simulink library "ammclib_bam_S32K3xx"  (R2016a)
(part 27 of 50)

      |           warning('Natural frequency f0 must be positive.');
      |         end
      |         if (iksi<=0)
      |           warning('Current loop attenuation must be positive.');
      |         end
      |         if (iksi>1)
      |           warning('Current loop attenuation must not exceed 1.');
      |         end
      |         pgain=12.56637061435917*iksi*if0;
      |         igain=39.47841760435743*if0*if0;
      |         if strcmp(intmethod,'Forward Rectangular')
      |           cc1=pgain;
      |           cc2=-pgain+igain*SampleTime;
      |         else
      |           if strcmp(intmethod,'Backward Rectangular')
      |             cc1=pgain+igain*SampleTime;
      |             cc2=-pgain;
      |           else
      |             cc1=pgain+igain*SampleTime*0.5;
      |             cc2=-pgain+igain*SampleTime*0.5;
      |           end
      |         end
      |         fltCC1sc=cc1;
      |         fltCC2sc=cc2;
      |         fltLowerLimit=-1000000.0;
      |         fltUpperLimit=1000000.0;
      |         fltC1=SampleTime*0.5;
      |         if isnan(fltCC1sc)
      |           if ~strcmp(fltCC1sc_bkup,'0')
      |             set_param(gcb,'fltCC1sc','0');
      |           end
      |         else
      |           tmps=num2str(fltCC1sc);
      |           if ~strcmp(fltCC1sc_bkup,tmps)
      |             set_param(gcb,'fltCC1sc',tmps);
      |           end
      |         end
      |         if isnan(fltCC2sc)
      |           if ~strcmp(fltCC2sc_bkup,'0')
      |             set_param(gcb,'fltCC2sc','0');
      |           end
      |         else
      |           tmps=num2str(fltCC2sc);
      |           if ~strcmp(fltCC2sc_bkup,tmps)
      |             set_param(gcb,'fltCC2sc',tmps);
      |           end
      |         end
      |         if isnan(fltUpperLimit)
      |           if ~strcmp(fltUpperLimit_bkup,'0')
      |             set_param(gcb,'fltUpperLimit','0');
      |           end
      |         else
      |           tmps=num2str(fltUpperLimit);
      |           if ~strcmp(fltUpperLimit_bkup,tmps)
      |             set_param(gcb,'fltUpperLimit',tmps);
      |           end
      |         end
      |         if isnan(fltLowerLimit)
      |           if ~strcmp(fltLowerLimit_bkup,'0')
      |             set_param(gcb,'fltLowerLimit','0');
      |           end
      |         else
      |           tmps=num2str(fltLowerLimit);
      |           if ~strcmp(fltLowerLimit_bkup,tmps)
      |             set_param(gcb,'fltLowerLimit',tmps);
      |           end
      |         end
      |         if isnan(fltC1)
      |           if ~strcmp(fltC1_bkup,'0')
      |             set_param(gcb,'fltC1','0');
      |           end
      |         else
      |           tmps=num2str(fltC1);
      |           if ~strcmp(fltC1_bkup,tmps)
      |             set_param(gcb,'fltC1',tmps);
      |           end
      |         end
      |       end
      |     end
      |   catch
      |    warning(['Sample time cannot be calculated for the block ' gcb])
      |   end
      | end
      mask DialogControl timeHint Prompt: Note: Implementation parameters cannot be calculated yet because the block's inherited sample time is unknown. Simulink will update the sample time when you run the simulation.
      mask Display:
      | color('black');
      | pos = get_param(gcb, 'Position');
      | width = pos(3) - pos(1);
      | height = pos(4) - pos(2);
      | tX=width/2;
      | tY=height - 25;
      | color('black');
      | text(tX,tY, 'AMCLIB_TrackObsrv_FLT', 'horizontalAlignment', 'center');
      | if showStates == 2
      |   color('red');
      |   text(tX,tY - 20, ['debugging mode' char(13) char(10) '(limited performance)'], 'horizontalAlignment', 'center');
      | end
  AMCLIB_Windmilling_FLT : Subsystem  StartFcn=|  TreatAsAtomicUnit=on  mask(AMCLIB_Windmilling_FLT){showStates=Hide (faster execution), SampleTime=-1, if0=350, iksi=1, ADCMaxError=0.002, autoCalcEn=on, fltADCMaxError=0, fltCC1sc=0, fltCC2sc=0, fltUpperLimit=0, fltLowerLimit=0, fltC1=0, SampleTime_1=NaN}
      | ts=get_param(gcb,'CompiledSampleTime');
      | if iscell(ts)
      |   ts=ts{1};
      |   if iscell(ts)
      |     ts=ts{1};
      |   end
      | end
      | ts=ts(1);
      | set_param(gcb,'SampleTime_1',num2str(ts));
      | p=Simulink.Mask.get(gcb);
      | hintText=p.getDialogControl('timeHint');
      | SampleTime=Simulink.data.evalinGlobal(bdroot,get_param(gcb,'SampleTime'));
      | p=Simulink.Mask.get(gcb);
      | autoCalcEn=get_param(gcb,'autoCalcEn');
      | if strcmp(autoCalcEn,'on')
      |   if SampleTime==-1
      |     hintText.Prompt='Caution: Implementation parameters depend on inherited sample time. Make sure that the sample time of the block''s inputs corresponds to the sampling period in the target application.';
      |   else
      |     hintText.Prompt='Caution: Implementation parameters depend on the sample time. Make sure that the simulation time step corresponds to the sampling period in the target application.';
      |   end
      |   SampleTime=ts;
      |   fltADCMaxError_bkup=get_param(gcb,'fltADCMaxError');
      |   fltCC1sc_bkup=get_param(gcb,'fltCC1sc');
      |   fltCC2sc_bkup=get_param(gcb,'fltCC2sc');
      |   fltUpperLimit_bkup=get_param(gcb,'fltUpperLimit');
      |   fltLowerLimit_bkup=get_param(gcb,'fltLowerLimit');
      |   fltC1_bkup=get_param(gcb,'fltC1');
      |   if0=Simulink.data.evalinGlobal(bdroot,get_param(gcb,'if0'));
      |   iksi=Simulink.data.evalinGlobal(bdroot,get_param(gcb,'iksi'));
      |   ADCMaxError=Simulink.data.evalinGlobal(bdroot,get_param(gcb,'ADCMaxError'));
      |   if (if0<=0)
      |     warning('Natural frequency f0 must be positive.');
      |   end
      |   if (iksi<=0)
      |     warning('Feedback loop attenuation must be positive.');
      |   end
      |   if (iksi>1)
      |     warning('Feedback loop attenuation must not exceed 1.');
      |   end
      |   if (ADCMaxError<=0)
      |     warning('fltADCMaxError must be positive.');
      |   end
      |   fltADCMaxError=ADCMaxError;
      |   pgain=12.56637061435917*iksi*if0;
      |   igain=39.47841760435743*if0*if0;
      |   cc1=pgain+igain*SampleTime*0.5;
      |   cc2=-pgain+igain*SampleTime*0.5;
      |   fltCC1sc=cc1;
      |   fltCC2sc=cc2;
      |   fltLowerLimit=-1000000.0;
      |   fltUpperLimit=1000000.0;
      |   fltC1=SampleTime*0.5;
      |   if isnan(fltADCMaxError)
      |     if ~strcmp(fltADCMaxError_bkup,'0')
      |       set_param(gcb,'fltADCMaxError','0');
      |     end
      |   else
      |     tmps=num2str(fltADCMaxError);
      |     if ~strcmp(fltADCMaxError_bkup,tmps)
      |       set_param(gcb,'fltADCMaxError',tmps);
      |     end
      |   end
      |   if isnan(fltCC1sc)
      |     if ~strcmp(fltCC1sc_bkup,'0')
      |       set_param(gcb,'fltCC1sc','0');
      |     end
      |   else
      |     tmps=num2str(fltCC1sc);
      |     if ~strcmp(fltCC1sc_bkup,tmps)
      |       set_param(gcb,'fltCC1sc',tmps);
      |     end
      |   end
      |   if isnan(fltCC2sc)
      |     if ~strcmp(fltCC2sc_bkup,'0')
      |       set_param(gcb,'fltCC2sc','0');
      |     end
      |   else
      |     tmps=num2str(fltCC2sc);
      |     if ~strcmp(fltCC2sc_bkup,tmps)
      |       set_param(gcb,'fltCC2sc',tmps);
      |     end
      |   end
      |   if isnan(fltUpperLimit)
      |     if ~strcmp(fltUpperLimit_bkup,'0')
      |       set_param(gcb,'fltUpperLimit','0');
      |     end
      |   else
      |     tmps=num2str(fltUpperLimit);
      |     if ~strcmp(fltUpperLimit_bkup,tmps)
      |       set_param(gcb,'fltUpperLimit',tmps);
      |     end
      |   end
      |   if isnan(fltLowerLimit)
      |     if ~strcmp(fltLowerLimit_bkup,'0')
      |       set_param(gcb,'fltLowerLimit','0');
      |     end
      |   else
      |     tmps=num2str(fltLowerLimit);
      |     if ~strcmp(fltLowerLimit_bkup,tmps)
      |       set_param(gcb,'fltLowerLimit',tmps);
      |     end
      |   end
      |   if isnan(fltC1)
      |     if ~strcmp(fltC1_bkup,'0')
      |       set_param(gcb,'fltC1','0');
      |     end
      |   else
      |     tmps=num2str(fltC1);
      |     if ~strcmp(fltC1_bkup,tmps)
      |       set_param(gcb,'fltC1',tmps);
      |     end
      |   end
      | end
      mask prompts: showStates "Show internal states:"; SampleTime "Sample time (-1 for inherited):"; if0 "Feedback loop natural frequency f0 [Hz]:"; iksi "Feedback loop attenuation ξ:"; ADCMaxError "Maximum differential offset error between any two
phases of the 3-phase voltage-sensing A/D converters [V]:"; autoCalcEn "Calculate implementation parameters from physical parameters"; fltADCMaxError "fltADCMaxError (Max. ADC differential offset error):"; fltCC1sc "fltCC1sc (GFLIB_ControllerPIrAW - CC1 coefficient):"; fltCC2sc "fltCC2sc (GFLIB_ControllerPIrAW - CC2 coefficient):"; fltUpperLimit "fltUpperLimit (GFLIB_ControllerPIrAW - upper Limit of the controller):"; fltLowerLimit "fltLowerLimit (GFLIB_ControllerPIrAW - lower Limit of the controller):"; fltC1 "fltC1 (GFLIB_IntegratorTR - integrator coefficient):"; SampleTime_1 "Discrete sample time:"
      mask help: PMSM Windmilling in single precision floating-point implementation. This function detects spontaneous rotation of an unpowered 3-phase PMSM by measuring the generated back electromotive force. Output u32Lock represents the return value of the C function (0 = undecided, 1 = spinning, 2 = stopped). Transition from 0 to 1 on the u32Lock output can be taken as a reset signal for the following AMCLIB_TrackObsrv_FLT block to synchronize the sensorless FOC loop with a freewheeling motor. Refer to the AMMCLIB User's Guide for further details.
      mask init:
      | ddName = get_param(bdroot,'DataDictionary');
      | if length(ddName)==0
      |   set_param(bdroot,'DataDictionary','ammclib_types.sldd');
      | else
      |   dd = Simulink.data.dictionary.open(ddName);
      |   data = getSection(dd,'Design Data');
      |   if ~exist(data,'SWLIBS_2Syst_F16')
      |     addDataSource(dd,'ammclib_types.sldd');
      |     saveChanges(dd);
      |   end
      | end
      | 
      | if showStates == 1
      |   % hidden state variables
      |   if strcmp(get_param([gcb '/fltADCMaxError'], 'BlockType'), 'Inport')
      |     posblk = get_param(gcb, 'Position');
      | 
      |     pos = get_param([gcb, '/fltADCMaxError'], 'Position');
      |     orient = get_param([gcb, '/fltADCMaxError'], 'Orientation');
      |     delete_block([gcb, '/fltADCMaxError']);
      |     add_block('built-in/Ground', [gcb, '/fltADCMaxError'], 'Position', pos, 'Orientation', orient);
      | 
      |     pos = get_param([gcb, '/fltCC1sc'], 'Position');
      |     orient = get_param([gcb, '/fltCC1sc'], 'Orientation');
      |     delete_block([gcb, '/fltCC1sc']);
      |     add_block('built-in/Ground', [gcb, '/fltCC1sc'], 'Position', pos, 'Orientation', orient);
      | 
      |     pos = get_param([gcb, '/fltCC2sc'], 'Position');
      |     orient = get_param([gcb, '/fltCC2sc'], 'Orientation');
      |     delete_block([gcb, '/fltCC2sc']);
      |     add_block('built-in/Ground', [gcb, '/fltCC2sc'], 'Position', pos, 'Orientation', orient);
      | 
      |     pos = get_param([gcb, '/fltUpperLimit'], 'Position');
      |     orient = get_param([gcb, '/fltUpperLimit'], 'Orientation');
      |     delete_block([gcb, '/fltUpperLimit']);
      |     add_block('built-in/Ground', [gcb, '/fltUpperLimit'], 'Position', pos, 'Orientation', orient);
      | 
      |     pos = get_param([gcb, '/fltLowerLimit'], 'Position');
      |     orient = get_param([gcb, '/fltLowerLimit'], 'Orientation');
      |     delete_block([gcb, '/fltLowerLimit']);
      |     add_block('built-in/Ground', [gcb, '/fltLowerLimit'], 'Position', pos, 'Orientation', orient);
      | 
      |     pos = get_param([gcb, '/fltC1'], 'Position');
      |     orient = get_param([gcb, '/fltC1'], 'Orientation');
      |     delete_block([gcb, '/fltC1']);
      |     add_block('built-in/Ground', [gcb, '/fltC1'], 'Position', pos, 'Orientation', orient);
      | 
      |     pos = get_param([gcb, '/fltAccPI'], 'Position');
      |     orient = get_param([gcb, '/fltAccPI'], 'Orientation');
      |     delete_block([gcb, '/fltAccPI']);
      |     add_block('built-in/Ground', [gcb, '/fltAccPI'], 'Position', pos, 'Orientation', orient);
      | 
      |     pos = get_param([gcb, '/fltInErrK1'], 'Position');
      |     orient = get_param([gcb, '/fltInErrK1'], 'Orientation');
      |     delete_block([gcb, '/fltInErrK1']);
      |     add_block('built-in/Ground', [gcb, '/fltInErrK1'], 'Position', pos, 'Orientation', orient);
      | 
      |     pos = get_param([gcb, '/fltState'], 'Position');
      |     orient = get_param([gcb, '/fltState'], 'Orientation');
      |     delete_block([gcb, '/fltState']);
      |     add_block('built-in/Ground', [gcb, '/fltState'], 'Position', pos, 'Orientation', orient);
      | 
      |     pos = get_param([gcb, '/fltInK1'], 'Position');
      |     orient = get_param([gcb, '/fltInK1'], 'Orientation');
      |     delete_block([gcb, '/fltInK1']);
      |     add_block('built-in/Ground', [gcb, '/fltInK1'], 'Position', pos, 'Orientation', orient);
      | 
      | 
      |     pmask=Simulink.Mask.get(gcb);
      |     pctrl=pmask.getParameter('SampleTime');
      |     pctrl.set('TypeOptions',{'pUabcIn/SampleTime'});
      | 
      |     pos = get_param([gcb '/fltAccPI_Out'], 'Position');
      |     orient = get_param([gcb '/fltAccPI_Out'], 'Orientation');
      |     delete_block([gcb '/fltAccPI_Out']);
      |     add_block('built-in/Terminator', [gcb '/fltAccPI_Out'], 'Position', pos, 'Orientation', orient);
      | 
      |     pos = get_param([gcb '/fltInErrK1_Out'], 'Position');
      |     orient = get_param([gcb '/fltInErrK1_Out'], 'Orientation');
      |     delete_block([gcb '/fltInErrK1_Out']);
      |     add_block('built-in/Terminator', [gcb '/fltInErrK1_Out'], 'Position', pos, 'Orientation', orient);
      | 
      |     pos = get_param([gcb '/fltState_Out'], 'Position');
      |     orient = get_param([gcb '/fltState_Out'], 'Orientation');
      |     delete_block([gcb '/fltState_Out']);
      |     add_block('built-in/Terminator', [gcb '/fltState_Out'], 'Position', pos, 'Orientation', orient);
      | 
      |     pos = get_param([gcb '/fltInK1_Out'], 'Position');
      |     orient = get_param([gcb '/fltInK1_Out'], 'Orientation');
      |     delete_block([gcb '/fltInK1_Out']);
      |     add_block('built-in/Terminator', [gcb '/fltInK1_Out'], 'Position', pos, 'Orientation', orient);
      | 
      |     set_param([gcb '/pUabcIn'], 'Port', '1');
      | 
      |     tmpOutCnt=0;
      |     tmpOutCnt=tmpOutCnt+1;
      |     set_param([gcb '/u32Lock'], 'Port', num2str(tmpOutCnt));
      |     tmpOutCnt=tmpOutCnt+1;
      |     set_param([gcb '/pPosEst'], 'Port', num2str(tmpOutCnt));
      |     tmpOutCnt=tmpOutCnt+1;
      |     set_param([gcb '/pVelocityEst'], 'Port', num2str(tmpOutCnt));
      | 
      |     autoCalcEn=get_param(gcb,'autoCalcEn');
      |     if strcmp(autoCalcEn,'on')
      |       set_param(gcb,'MaskEnables',{'on','on','on','on','on','on','on','on','on','on','on','on','off'});
      |     else
      |       set_param(gcb,'MaskEnables',{'on','on','off','off','off','on','on','on','on','on','on','on','off'});
      |     end
      | 
      |     if (posblk(4) - posblk(2)) > 100
      |       height = 100;
      |       set_param(gcb,'Position',[posblk(1), posblk(2), posblk(3), posblk(2)+height])
      |     end
      |   end
      | else
      |   % shown state variables
      |   if strcmp(get_param([gcb '/fltADCMaxError'], 'BlockType'), 'Ground')
      |     posblk = get_param(gcb, 'Position');
      | 
      |     pos = get_param([gcb, '/fltADCMaxError'], 'Position');
      |     orient = get_param([gcb, '/fltADCMaxError'], 'Orientation');
      |     delete_block([gcb, '/fltADCMaxError']);
      |     add_block('built-in/Inport', [gcb, '/fltADCMaxError'], 'Position', pos, 'Orientation', orient, 'OutDataTypeStr', 'single');
      | 
      |     pos = get_param([gcb, '/fltCC1sc'], 'Position');
      |     orient = get_param([gcb, '/fltCC1sc'], 'Orientation');
      |     delete_block([gcb, '/fltCC1sc']);
      |     add_block('built-in/Inport', [gcb, '/fltCC1sc'], 'Position', pos, 'Orientation', orient, 'OutDataTypeStr', 'single');
      | 
      |     pos = get_param([gcb, '/fltCC2sc'], 'Position');
      |     orient = get_param([gcb, '/fltCC2sc'], 'Orientation');
      |     delete_block([gcb, '/fltCC2sc']);
      |     add_block('built-in/Inport', [gcb, '/fltCC2sc'], 'Position', pos, 'Orientation', orient, 'OutDataTypeStr', 'single');
      | 
      |     pos = get_param([gcb, '/fltUpperLimit'], 'Position');
      |     orient = get_param([gcb, '/fltUpperLimit'], 'Orientation');
      |     delete_block([gcb, '/fltUpperLimit']);
      |     add_block('built-in/Inport', [gcb, '/fltUpperLimit'], 'Position', pos, 'Orientation', orient, 'OutDataTypeStr', 'single');
      | 
      |     pos = get_param([gcb, '/fltLowerLimit'], 'Position');
      |     orient = get_param([gcb, '/fltLowerLimit'], 'Orientation');
      |     delete_block([gcb, '/fltLowerLimit']);
      |     add_block('built-in/Inport', [gcb, '/fltLowerLimit'], 'Position', pos, 'Orientation', orient, 'OutDataTypeStr', 'single');
      | 
      |     pos = get_param([gcb, '/fltC1'], 'Position');
      |     orient = get_param([gcb, '/fltC1'], 'Orientation');
      |     delete_block([gcb, '/fltC1']);
      |     add_block('built-in/Inport', [gcb, '/fltC1'], 'Position', pos, 'Orientation', orient, 'OutDataTypeStr', 'single');
      | 
      |     pos = get_param([gcb, '/fltAccPI'], 'Position');
      |     orient = get_param([gcb, '/fltAccPI'], 'Orientation');
      |     delete_block([gcb, '/fltAccPI']);
      |     add_block('built-in/Inport', [gcb, '/fltAccPI'], 'Position', pos, 'Orientation', orient, 'OutDataTypeStr', 'single');
      | 
      |     pos = get_param([gcb, '/fltInErrK1'], 'Position');
      |     orient = get_param([gcb, '/fltInErrK1'], 'Orientation');
      |     delete_block([gcb, '/fltInErrK1']);
      |     add_block('built-in/Inport', [gcb, '/fltInErrK1'], 'Position', pos, 'Orientation', orient, 'OutDataTypeStr', 'single');
      | 
      |     pos = get_param([gcb, '/fltState'], 'Position');
      |     orient = get_param([gcb, '/fltState'], 'Orientation');
      |     delete_block([gcb, '/fltState']);
      |     add_block('built-in/Inport', [gcb, '/fltState'], 'Position', pos, 'Orientation', orient, 'OutDataTypeStr', 'single');
      | 
      |     pos = get_param([gcb, '/fltInK1'], 'Position');
      |     orient = get_param([gcb, '/fltInK1'], 'Orientation');
      |     delete_block([gcb, '/fltInK1']);
      |     add_block('built-in/Inport', [gcb, '/fltInK1'], 'Position', pos, 'Orientation', orient, 'OutDataTypeStr', 'single');
      | 
      | 
      | 
      |     pos = get_param([gcb '/fltAccPI_Out'], 'Position');
      |     orient = get_param([gcb '/fltAccPI_Out'], 'Orientation');
      |     delete_block([gcb '/fltAccPI_Out']);
      |     add_block('built-in/Outport', [gcb '/fltAccPI_Out'], 'Position', pos, 'Orientation', orient);
      | 
      |     pos = get_param([gcb '/fltInErrK1_Out'], 'Position');
      |     orient = get_param([gcb '/fltInErrK1_Out'], 'Orientation');
      |     delete_block([gcb '/fltInErrK1_Out']);
      |     add_block('built-in/Outport', [gcb '/fltInErrK1_Out'], 'Position', pos, 'Orientation', orient);
      | 
      |     pos = get_param([gcb '/fltState_Out'], 'Position');
      |     orient = get_param([gcb '/fltState_Out'], 'Orientation');
      |     delete_block([gcb '/fltState_Out']);
      |     add_block('built-in/Outport', [gcb '/fltState_Out'], 'Position', pos, 'Orientation', orient);
      | 
      |     pos = get_param([gcb '/fltInK1_Out'], 'Position');
      |     orient = get_param([gcb '/fltInK1_Out'], 'Orientation');
      |     delete_block([gcb '/fltInK1_Out']);
      |     add_block('built-in/Outport', [gcb '/fltInK1_Out'], 'Position', pos, 'Orientation', orient);
      | 
      | 
      |     pmask=Simulink.Mask.get(gcb);
      |     pctrl=pmask.getParameter('SampleTime');
      |     pctrl.set('TypeOptions',{'pUabcIn/SampleTime','fltADCMaxError/SampleTime','fltCC1sc/SampleTime','fltCC2sc/SampleTime','fltUpperLimit/SampleTime','fltLowerLimit/SampleTime','fltC1/SampleTime','fltAccPI/SampleTime','fltInErrK1/SampleTime','fltState/SampleTime','fltInK1/SampleTime'});
      | 
      |     set_param([gcb '/pUabcIn'], 'Port', '1');
      |     set_param([gcb '/fltADCMaxError'], 'Port', '2');
      |     set_param([gcb '/fltCC1sc'], 'Port', '3');
      |     set_param([gcb '/fltCC2sc'], 'Port', '4');
      |     set_param([gcb '/fltUpperLimit'], 'Port', '5');
      |     set_param([gcb '/fltLowerLimit'], 'Port', '6');
      |     set_param([gcb '/fltC1'], 'Port', '7');
      |     set_param([gcb '/fltAccPI'], 'Port', '8');
      |     set_param([gcb '/fltInErrK1'], 'Port', '9');
      |     set_param([gcb '/fltState'], 'Port', '10');
      |     set_param([gcb '/fltInK1'], 'Port', '11');
      | 
      |     tmpOutCnt=0;
      |     tmpOutCnt=tmpOutCnt+1;
      |     set_param([gcb '/u32Lock'], 'Port', num2str(tmpOutCnt));
      |     tmpOutCnt=tmpOutCnt+1;
      |     set_param([gcb '/pPosEst'], 'Port', num2str(tmpOutCnt));
      |     tmpOutCnt=tmpOutCnt+1;
      |     set_param([gcb '/pVelocityEst'], 'Port', num2str(tmpOutCnt));
      |     tmpOutCnt=tmpOutCnt+1;
      |     set_param([gcb '/fltAccPI_Out'], 'Port', num2str(tmpOutCnt));
      |     tmpOutCnt=tmpOutCnt+1;
      |     set_param([gcb '/fltInErrK1_Out'], 'Port', num2str(tmpOutCnt));
      |     tmpOutCnt=tmpOutCnt+1;
      |     set_param([gcb '/fltState_Out'], 'Port', num2str(tmpOutCnt));
      |     tmpOutCnt=tmpOutCnt+1;
      |     set_param([gcb '/fltInK1_Out'], 'Port', num2str(tmpOutCnt));
      | 
      |     set_param(gcb,'MaskEnables',{'on','on','off','off','off','off','off','off','off','off','off','off','off'});
      | 
      |     if (posblk(4) - posblk(2)) < 300
      |       height = 300;
      |       set_param(gcb,'Position',[posblk(1), posblk(2), posblk(3), posblk(2)+height])
      |     end
      |   end
      | end
      settings: RTWSystemCode=Inline
      mask Help: web([fileparts(which('ammclib_bam_S32K3xx.slx')) '/../doc/S32K3XXMCLUG.pdf'], '-browser')
      mask TypeOptions showStates: Hide (faster execution) | Show (allows debugging; connect feedback loops manually)
      mask Callback showStates:
      | maskStr=get_param(gcb,'showStates');
      | if strcmp(maskStr,'Hide (faster execution)')
      |   if strcmp(get_param([gcb '/fltADCMaxError'], 'BlockType'), 'Inport')
      |     autoCalcEn=get_param(gcb,'autoCalcEn');
      |     if strcmp(autoCalcEn,'on')
      |       set_param(gcb,'MaskEnables',{'on','on','on','on','on','on','on','on','on','on','on','on','off'});
      |     else
      |       set_param(gcb,'MaskEnables',{'on','on','off','off','off','on','on','on','on','on','on','on','off'});
      |     end
      |   end
      | else
      |   if strcmp(get_param([gcb '/fltADCMaxError'], 'BlockType'), 'Ground')
      |     set_param(gcb,'MaskEnables',{'on','on','off','off','off','off','off','off','off','off','off','off','off'});
      |   end
      | end
      mask TypeOptions SampleTime: pUabcIn/SampleTime
      mask Callback SampleTime:
      | p=Simulink.Mask.get(gcb);
      | hintText=p.getDialogControl('timeHint');
      | SampleTime=Simulink.data.evalinGlobal(bdroot,get_param(gcb,'SampleTime'));
      | SampleTime_1=str2double(get_param(gcb,'SampleTime_1'));
      | if (((SampleTime==-1) && (~contains(hintText.Prompt,'inherited'))) || ...
      |     ((SampleTime~=-1) && contains(hintText.Prompt,'inherited')) || ...
      |     ((SampleTime~=-1) && (SampleTime_1~=SampleTime)) || ...
      |     ((SampleTime_1~=-1) && contains(hintText.Prompt,'yet')))
      |   if ((SampleTime==-1) && (~contains(hintText.Prompt,'inherited')))
      |     set_param(gcb,'SampleTime_1',num2str(NaN));
      |     SampleTime_1=NaN;
      |   end
      |   if (SampleTime~=-1)
      |     set_param(gcb,'SampleTime_1',num2str(SampleTime));
      |     SampleTime_1=SampleTime;
      |   end
      |   autoCalcEn=get_param(gcb,'autoCalcEn');
      |   if strcmp(autoCalcEn,'on')
      |     p=Simulink.Mask.get(gcb);
      |     hintText=p.getDialogControl('timeHint');
      |     if SampleTime==-1
      |       SampleTime=SampleTime_1;
      |       if isnan(SampleTime)
      |         hintText.Prompt='Note: Implementation parameters cannot be calculated yet because the block''s inherited sample time is unknown. Simulink will update the sample time when you run the simulation.';
      |       else
      |         hintText.Prompt='Caution: Implementation parameters depend on inherited sample time. Make sure that the sample time of the block''s inputs corresponds to the sampling period in the target application.';
      |       end
      |     else
      |       hintText.Prompt='Caution: Implementation parameters depend on the sample time. Make sure that the simulation time step corresponds to the sampling period in the target application.';
      |     end
      |     fltADCMaxError_bkup=get_param(gcb,'fltADCMaxError');
      |     fltCC1sc_bkup=get_param(gcb,'fltCC1sc');
      |     fltCC2sc_bkup=get_param(gcb,'fltCC2sc');
      |     fltUpperLimit_bkup=get_param(gcb,'fltUpperLimit');
      |     fltLowerLimit_bkup=get_param(gcb,'fltLowerLimit');
      |     fltC1_bkup=get_param(gcb,'fltC1');
      |     if0=Simulink.data.evalinGlobal(bdroot,get_param(gcb,'if0'));
      |     iksi=Simulink.data.evalinGlobal(bdroot,get_param(gcb,'iksi'));
      |     ADCMaxError=Simulink.data.evalinGlobal(bdroot,get_param(gcb,'ADCMaxError'));
      |     if (if0<=0)
      |       warning('Natural frequency f0 must be positive.');
      |     end
      |     if (iksi<=0)
      |       warning('Feedback loop attenuation must be positive.');
      |     end
      |     if (iksi>1)
      |       warning('Feedback loop attenuation must not exceed 1.');
      |     end
      |     if (ADCMaxError<=0)
      |       warning('fltADCMaxError must be positive.');
      |     end
      |     fltADCMaxError=ADCMaxError;
      |     pgain=12.56637061435917*iksi*if0;
      |     igain=39.47841760435743*if0*if0;
      |     cc1=pgain+igain*SampleTime*0.5;
      |     cc2=-pgain+igain*SampleTime*0.5;
      |     fltCC1sc=cc1;
      |     fltCC2sc=cc2;
      |     fltLowerLimit=-1000000.0;
      |     fltUpperLimit=1000000.0;
      |     fltC1=SampleTime*0.5;
      |     if isnan(fltADCMaxError)
      |       if ~strcmp(fltADCMaxError_bkup,'0')
      |         set_param(gcb,'fltADCMaxError','0');
      |       end
      |     else
      |       tmps=num2str(fltADCMaxError);
      |       if ~strcmp(fltADCMaxError_bkup,tmps)
      |         set_param(gcb,'fltADCMaxError',tmps);
      |       end
      |     end
      |     if isnan(fltCC1sc)
      |       if ~strcmp(fltCC1sc_bkup,'0')
      |         set_param(gcb,'fltCC1sc','0');
      |       end
      |     else
      |       tmps=num2str(fltCC1sc);
      |       if ~strcmp(fltCC1sc_bkup,tmps)
      |         set_param(gcb,'fltCC1sc',tmps);
      |       end
      |     end
      |     if isnan(fltCC2sc)
      |       if ~strcmp(fltCC2sc_bkup,'0')
      |         set_param(gcb,'fltCC2sc','0');
      |       end
      |     else
      |       tmps=num2str(fltCC2sc);
      |       if ~strcmp(fltCC2sc_bkup,tmps)
      |         set_param(gcb,'fltCC2sc',tmps);
      |       end
      |     end
      |     if isnan(fltUpperLimit)
      |       if ~strcmp(fltUpperLimit_bkup,'0')
      |         set_param(gcb,'fltUpperLimit','0');
      |       end
      |     else
      |       tmps=num2str(fltUpperLimit);
      |       if ~strcmp(fltUpperLimit_bkup,tmps)
      |         set_param(gcb,'fltUpperLimit',tmps);
      |       end
      |     end
      |     if isnan(fltLowerLimit)
      |       if ~strcmp(fltLowerLimit_bkup,'0')
      |         set_param(gcb,'fltLowerLimit','0');
      |       end
      |     else
      |       tmps=num2str(fltLowerLimit);
      |       if ~strcmp(fltLowerLimit_bkup,tmps)
      |         set_param(gcb,'fltLowerLimit',tmps);
      |       end
      |     end
      |     if isnan(fltC1)
      |       if ~strcmp(fltC1_bkup,'0')
      |         set_param(gcb,'fltC1','0');
      |       end
      |     else
      |       tmps=num2str(fltC1);
      |       if ~strcmp(fltC1_bkup,tmps)
      |         set_param(gcb,'fltC1',tmps);
      |       end
      |     end
      |   end
      | end
      mask Callback if0:
      | autoCalcEn=get_param(gcb,'autoCalcEn');
      | if strcmp(autoCalcEn,'on')
      |   SampleTime=Simulink.data.evalinGlobal(bdroot,get_param(gcb,'SampleTime'));
      |   if (SampleTime==-1)
      |     SampleTime=str2double(get_param(gcb,'SampleTime_1'));
      |   end
      |   fltADCMaxError_bkup=get_param(gcb,'fltADCMaxError');
      |   fltCC1sc_bkup=get_param(gcb,'fltCC1sc');
      |   fltCC2sc_bkup=get_param(gcb,'fltCC2sc');
      |   fltUpperLimit_bkup=get_param(gcb,'fltUpperLimit');
      |   fltLowerLimit_bkup=get_param(gcb,'fltLowerLimit');
      |   fltC1_bkup=get_param(gcb,'fltC1');
      |   if0=Simulink.data.evalinGlobal(bdroot,get_param(gcb,'if0'));
      |   iksi=Simulink.data.evalinGlobal(bdroot,get_param(gcb,'iksi'));
      |   ADCMaxError=Simulink.data.evalinGlobal(bdroot,get_param(gcb,'ADCMaxError'));
      |   if (if0<=0)
      |     warning('Natural frequency f0 must be positive.');
      |   end
      |   if (iksi<=0)
      |     warning('Feedback loop attenuation must be positive.');
      |   end
      |   if (iksi>1)
      |     warning('Feedback loop attenuation must not exceed 1.');
      |   end
      |   if (ADCMaxError<=0)
      |     warning('fltADCMaxError must be positive.');
      |   end
      |   fltADCMaxError=ADCMaxError;
      |   pgain=12.56637061435917*iksi*if0;
      |   igain=39.47841760435743*if0*if0;
      |   cc1=pgain+igain*SampleTime*0.5;
      |   cc2=-pgain+igain*SampleTime*0.5;
      |   fltCC1sc=cc1;
      |   fltCC2sc=cc2;
      |   fltLowerLimit=-1000000.0;
      |   fltUpperLimit=1000000.0;
      |   fltC1=SampleTime*0.5;
      |   if isnan(fltADCMaxError)
      |     if ~strcmp(fltADCMaxError_bkup,'0')
      |       set_param(gcb,'fltADCMaxError','0');
      |     end
      |   else
      |     tmps=num2str(fltADCMaxError);
      |     if ~strcmp(fltADCMaxError_bkup,tmps)
      |       set_param(gcb,'fltADCMaxError',tmps);
      |     end
      |   end
      |   if isnan(fltCC1sc)
      |     if ~strcmp(fltCC1sc_bkup,'0')
      |       set_param(gcb,'fltCC1sc','0');
      |     end
      |   else
      |     tmps=num2str(fltCC1sc);
      |     if ~strcmp(fltCC1sc_bkup,tmps)
      |       set_param(gcb,'fltCC1sc',tmps);
      |     end
      |   end
      |   if isnan(fltCC2sc)
      |     if ~strcmp(fltCC2sc_bkup,'0')
      |       set_param(gcb,'fltCC2sc','0');
      |     end
      |   else
      |     tmps=num2str(fltCC2sc);
      |     if ~strcmp(fltCC2sc_bkup,tmps)
      |       set_param(gcb,'fltCC2sc',tmps);
      |     end
      |   end
      |   if isnan(fltUpperLimit)
      |     if ~strcmp(fltUpperLimit_bkup,'0')
      |       set_param(gcb,'fltUpperLimit','0');
      |     end
      |   else
      |     tmps=num2str(fltUpperLimit);
      |     if ~strcmp(fltUpperLimit_bkup,tmps)
      |       set_param(gcb,'fltUpperLimit',tmps);
      |     end
      |   end
      |   if isnan(fltLowerLimit)
      |     if ~strcmp(fltLowerLimit_bkup,'0')
      |       set_param(gcb,'fltLowerLimit','0');
      |     end
      |   else
      |     tmps=num2str(fltLowerLimit);
      |     if ~strcmp(fltLowerLimit_bkup,tmps)
      |       set_param(gcb,'fltLowerLimit',tmps);
      |     end
      |   end
      |   if isnan(fltC1)
      |     if ~strcmp(fltC1_bkup,'0')
      |       set_param(gcb,'fltC1','0');
      |     end
      |   else
      |     tmps=num2str(fltC1);
      |     if ~strcmp(fltC1_bkup,tmps)
      |       set_param(gcb,'fltC1',tmps);
      |     end
      |   end
      | end
      mask Callback iksi:
      | autoCalcEn=get_param(gcb,'autoCalcEn');
      | if strcmp(autoCalcEn,'on')
      |   SampleTime=Simulink.data.evalinGlobal(bdroot,get_param(gcb,'SampleTime'));
      |   if (SampleTime==-1)
      |     SampleTime=str2double(get_param(gcb,'SampleTime_1'));
      |   end
      |   fltADCMaxError_bkup=get_param(gcb,'fltADCMaxError');
      |   fltCC1sc_bkup=get_param(gcb,'fltCC1sc');
      |   fltCC2sc_bkup=get_param(gcb,'fltCC2sc');
      |   fltUpperLimit_bkup=get_param(gcb,'fltUpperLimit');
      |   fltLowerLimit_bkup=get_param(gcb,'fltLowerLimit');
      |   fltC1_bkup=get_param(gcb,'fltC1');
      |   if0=Simulink.data.evalinGlobal(bdroot,get_param(gcb,'if0'));
      |   iksi=Simulink.data.evalinGlobal(bdroot,get_param(gcb,'iksi'));
      |   ADCMaxError=Simulink.data.evalinGlobal(bdroot,get_param(gcb,'ADCMaxError'));
      |   if (if0<=0)
      |     warning('Natural frequency f0 must be positive.');
      |   end
      |   if (iksi<=0)
      |     warning('Feedback loop attenuation must be positive.');
      |   end
      |   if (iksi>1)
      |     warning('Feedback loop attenuation must not exceed 1.');
      |   end
      |   if (ADCMaxError<=0)
      |     warning('fltADCMaxError must be positive.');
      |   end
      |   fltADCMaxError=ADCMaxError;
      |   pgain=12.56637061435917*iksi*if0;
      |   igain=39.47841760435743*if0*if0;
      |   cc1=pgain+igain*SampleTime*0.5;
      |   cc2=-pgain+igain*SampleTime*0.5;
      |   fltCC1sc=cc1;
      |   fltCC2sc=cc2;
      |   fltLowerLimit=-1000000.0;
      |   fltUpperLimit=1000000.0;
      |   fltC1=SampleTime*0.5;
      |   if isnan(fltADCMaxError)
      |     if ~strcmp(fltADCMaxError_bkup,'0')
      |       set_param(gcb,'fltADCMaxError','0');
      |     end
      |   else
      |     tmps=num2str(fltADCMaxError);
      |     if ~strcmp(fltADCMaxError_bkup,tmps)
      |       set_param(gcb,'fltADCMaxError',tmps);
      |     end
      |   end
      |   if isnan(fltCC1sc)
      |     if ~strcmp(fltCC1sc_bkup,'0')
      |       set_param(gcb,'fltCC1sc','0');
      |     end
      |   else
      |     tmps=num2str(fltCC1sc);
      |     if ~strcmp(fltCC1sc_bkup,tmps)
      |       set_param(gcb,'fltCC1sc',tmps);
      |     end
      |   end
      |   if isnan(fltCC2sc)
      |     if ~strcmp(fltCC2sc_bkup,'0')
      |       set_param(gcb,'fltCC2sc','0');
      |     end
      |   else
      |     tmps=num2str(fltCC2sc);
      |     if ~strcmp(fltCC2sc_bkup,tmps)
      |       set_param(gcb,'fltCC2sc',tmps);
      |     end
      |   end
      |   if isnan(fltUpperLimit)
      |     if ~strcmp(fltUpperLimit_bkup,'0')
      |       set_param(gcb,'fltUpperLimit','0');
      |     end
      |   else
      |     tmps=num2str(fltUpperLimit);
      |     if ~strcmp(fltUpperLimit_bkup,tmps)
      |       set_param(gcb,'fltUpperLimit',tmps);
      |     end
      |   end
      |   if isnan(fltLowerLimit)
      |     if ~strcmp(fltLowerLimit_bkup,'0')
      |       set_param(gcb,'fltLowerLimit','0');
      |     end
      |   else
      |     tmps=num2str(fltLowerLimit);
      |     if ~strcmp(fltLowerLimit_bkup,tmps)
      |       set_param(gcb,'fltLowerLimit',tmps);
      |     end
      |   end
      |   if isnan(fltC1)
      |     if ~strcmp(fltC1_bkup,'0')
      |       set_param(gcb,'fltC1','0');
      |     end
      |   else
      |     tmps=num2str(fltC1);
      |     if ~strcmp(fltC1_bkup,tmps)
      |       set_param(gcb,'fltC1',tmps);
      |     end
      |   end
      | end
      mask Callback ADCMaxError:
      | autoCalcEn=get_param(gcb,'autoCalcEn');
      | if strcmp(autoCalcEn,'on')
      |   SampleTime=Simulink.data.evalinGlobal(bdroot,get_param(gcb,'SampleTime'));
      |   if (SampleTime==-1)
      |     SampleTime=str2double(get_param(gcb,'SampleTime_1'));
      |   end
      |   fltADCMaxError_bkup=get_param(gcb,'fltADCMaxError');
      |   fltCC1sc_bkup=get_param(gcb,'fltCC1sc');
      |   fltCC2sc_bkup=get_param(gcb,'fltCC2sc');
      |   fltUpperLimit_bkup=get_param(gcb,'fltUpperLimit');
      |   fltLowerLimit_bkup=get_param(gcb,'fltLowerLimit');
      |   fltC1_bkup=get_param(gcb,'fltC1');
      |   if0=Simulink.data.evalinGlobal(bdroot,get_param(gcb,'if0'));
      |   iksi=Simulink.data.evalinGlobal(bdroot,get_param(gcb,'iksi'));
      |   ADCMaxError=Simulink.data.evalinGlobal(bdroot,get_param(gcb,'ADCMaxError'));
      |   if (if0<=0)
      |     warning('Natural frequency f0 must be positive.');
      |   end
      |   if (iksi<=0)
      |     warning('Feedback loop attenuation must be positive.');
      |   end
      |   if (iksi>1)
      |     warning('Feedback loop attenuation must not exceed 1.');
      |   end
      |   if (ADCMaxError<=0)
      |     warning('fltADCMaxError must be positive.');
      |   end
      |   fltADCMaxError=ADCMaxError;
      |   pgain=12.56637061435917*iksi*if0;
      |   igain=39.47841760435743*if0*if0;
      |   cc1=pgain+igain*SampleTime*0.5;
      |   cc2=-pgain+igain*SampleTime*0.5;
      |   fltCC1sc=cc1;
      |   fltCC2sc=cc2;
      |   fltLowerLimit=-1000000.0;
      |   fltUpperLimit=1000000.0;
      |   fltC1=SampleTime*0.5;
      |   if isnan(fltADCMaxError)
      |     if ~strcmp(fltADCMaxError_bkup,'0')
      |       set_param(gcb,'fltADCMaxError','0');
      |     end
      |   else
      |     tmps=num2str(fltADCMaxError);
      |     if ~strcmp(fltADCMaxError_bkup,tmps)
      |       set_param(gcb,'fltADCMaxError',tmps);
      |     end
      |   end
      |   if isnan(fltCC1sc)
      |     if ~strcmp(fltCC1sc_bkup,'0')
      |       set_param(gcb,'fltCC1sc','0');
      |     end
      |   else
      |     tmps=num2str(fltCC1sc);
      |     if ~strcmp(fltCC1sc_bkup,tmps)
      |       set_param(gcb,'fltCC1sc',tmps);
      |     end
      |   end
      |   if isnan(fltCC2sc)
      |     if ~strcmp(fltCC2sc_bkup,'0')
      |       set_param(gcb,'fltCC2sc','0');
      |     end
      |   else
      |     tmps=num2str(fltCC2sc);
      |     if ~strcmp(fltCC2sc_bkup,tmps)
      |       set_param(gcb,'fltCC2sc',tmps);
      |     end
      |   end
      |   if isnan(fltUpperLimit)
      |     if ~strcmp(fltUpperLimit_bkup,'0')
      |       set_param(gcb,'fltUpperLimit','0');
      |     end
      |   else
      |     tmps=num2str(fltUpperLimit);
      |     if ~strcmp(fltUpperLimit_bkup,tmps)
      |       set_param(gcb,'fltUpperLimit',tmps);
      |     end
      |   end
      |   if isnan(fltLowerLimit)
      |     if ~strcmp(fltLowerLimit_bkup,'0')
      |       set_param(gcb,'fltLowerLimit','0');
      |     end
      |   else
      |     tmps=num2str(fltLowerLimit);
      |     if ~strcmp(fltLowerLimit_bkup,tmps)
      |       set_param(gcb,'fltLowerLimit',tmps);
      |     end
      |   end
      |   if isnan(fltC1)
      |     if ~strcmp(fltC1_bkup,'0')
      |       set_param(gcb,'fltC1','0');
      |     end
      |   else
      |     tmps=num2str(fltC1);
      |     if ~strcmp(fltC1_bkup,tmps)
      |       set_param(gcb,'fltC1',tmps);
      |     end
      |   end
      | end
      mask Callback autoCalcEn:
      | maskStr=get_param(gcb,'showStates');
      | if strcmp(maskStr,'Hide (faster execution)')
      |   p=Simulink.Mask.get(gcb);
      |   autoCalcEn=get_param(gcb,'autoCalcEn');
      |   hintText=p.getDialogControl('timeHint');
      |   if strcmp(autoCalcEn,'on')
      |     param=p.getParameter('ADCMaxError');
      |     if strcmp(param.Enabled,'off')
      |       SampleTime=Simulink.data.evalinGlobal(bdroot,get_param(gcb,'SampleTime'));
      |       if SampleTime==-1
      |         SampleTime=str2double(get_param(gcb,'SampleTime_1'));
      |         if isnan(SampleTime)
      |           hintText.Prompt=['Note: Implementation parameters cannot be calculated yet because the block''s inherited sample time is unknown. Simulink will update the sample time when you run the simulation.'];
      |         else
      |           hintText.Prompt=['Caution: Implementation parameters depend on inherited sample time. Make sure that the sample time of the block''s inputs corresponds to the sampling period in the target application.'];
      |         end
      |       else
      |         hintText.Prompt='Caution: Implementation parameters depend on the sample time. Make sure that the simulation time step corresponds to the sampling period in the target application.';
      |       end
      |       p=Simulink.Mask.get(gcb);
      |       param=p.getParameter('if0');
      |       param.set('Enabled','on');
      |       param=p.getParameter('iksi');
      |       param.set('Enabled','on');
      |       param=p.getParameter('ADCMaxError');
      |       param.set('Enabled','on');
      |     else
      |       SampleTime=Simulink.data.evalinGlobal(bdroot,get_param(gcb,'SampleTime'));
      |       if SampleTime==-1
      |         SampleTime=str2double(get_param(gcb,'SampleTime_1'));
      |       end
      |     end
      |     fltADCMaxError_bkup=get_param(gcb,'fltADCMaxError');
      |     fltCC1sc_bkup=get_param(gcb,'fltCC1sc');
      |     fltCC2sc_bkup=get_param(gcb,'fltCC2sc');
      |     fltUpperLimit_bkup=get_param(gcb,'fltUpperLimit');
      |     fltLowerLimit_bkup=get_param(gcb,'fltLowerLimit');
      |     fltC1_bkup=get_param(gcb,'fltC1');
      |     if0=Simulink.data.evalinGlobal(bdroot,get_param(gcb,'if0'));
      |     iksi=Simulink.data.evalinGlobal(bdroot,get_param(gcb,'iksi'));
      |     ADCMaxError=Simulink.data.evalinGlobal(bdroot,get_param(gcb,'ADCMaxError'));
      |     if (if0<=0)
      |       warning('Natural frequency f0 must be positive.');
      |     end
      |     if (iksi<=0)
      |       warning('Feedback loop attenuation must be positive.');
      |     end
      |     if (iksi>1)
      |       warning('Feedback loop attenuation must not exceed 1.');
      |     end
      |     if (ADCMaxError<=0)
      |       warning('fltADCMaxError must be positive.');
      |     end
      |     fltADCMaxError=ADCMaxError;
      |     pgain=12.56637061435917*iksi*if0;
      |     igain=39.47841760435743*if0*if0;
      |     cc1=pgain+igain*SampleTime*0.5;
      |     cc2=-pgain+igain*SampleTime*0.5;
      |     fltCC1sc=cc1;
      |     fltCC2sc=cc2;
      |     fltLowerLimit=-1000000.0;
      |     fltUpperLimit=1000000.0;
      |     fltC1=SampleTime*0.5;
      |     if isnan(fltADCMaxError)
      |       if ~strcmp(fltADCMaxError_bkup,'0')
      |         set_param(gcb,'fltADCMaxError','0');
      |       end
      |     else
      |       tmps=num2str(fltADCMaxError);
      |       if ~strcmp(fltADCMaxError_bkup,tmps)
      |         set_param(gcb,'fltADCMaxError',tmps);
      |       end
      |     end
      |     if isnan(fltCC1sc)
      |       if ~strcmp(fltCC1sc_bkup,'0')
      |         set_param(gcb,'fltCC1sc','0');
      |       end
      |     else
      |       tmps=num2str(fltCC1sc);
      |       if ~strcmp(fltCC1sc_bkup,tmps)
      |         set_param(gcb,'fltCC1sc',tmps);
      |       end
      |     end
      |     if isnan(fltCC2sc)
      |       if ~strcmp(fltCC2sc_bkup,'0')
      |         set_param(gcb,'fltCC2sc','0');
      |       end
      |     else
      |       tmps=num2str(fltCC2sc);
      |       if ~strcmp(fltCC2sc_bkup,tmps)
      |         set_param(gcb,'fltCC2sc',tmps);
      |       end
      |     end
      |     if isnan(fltUpperLimit)
      |       if ~strcmp(fltUpperLimit_bkup,'0')
      |         set_param(gcb,'fltUpperLimit','0');
      |       end
      |     else
      |       tmps=num2str(fltUpperLimit);
      |       if ~strcmp(fltUpperLimit_bkup,tmps)
      |         set_param(gcb,'fltUpperLimit',tmps);
      |       end
      |     end
      |     if isnan(fltLowerLimit)
      |       if ~strcmp(fltLowerLimit_bkup,'0')
      |         set_param(gcb,'fltLowerLimit','0');
      |       end
      |     else
      |       tmps=num2str(fltLowerLimit);
      |       if ~strcmp(fltLowerLimit_bkup,tmps)
      |         set_param(gcb,'fltLowerLimit',tmps);
      |       end
      |     end
      |     if isnan(fltC1)
      |       if ~strcmp(fltC1_bkup,'0')
      |         set_param(gcb,'fltC1','0');
      |       end
      |     else
      |       tmps=num2str(fltC1);
      |       if ~strcmp(fltC1_bkup,tmps)
      |         set_param(gcb,'fltC1',tmps);
      |       end
      |     end
      |   else
      |     param=p.getParameter('ADCMaxError');
      |     if strcmp(param.Enabled,'on')
      |       hintText.Prompt='Caution: Implementation parameters are fixed.';
      |       p=Simulink.Mask.get(gcb);
      |       param=p.getParameter('if0');
      |       param.set('Enabled','off');
      |       param=p.getParameter('iksi');
      |       param.set('Enabled','off');
      |       param=p.getParameter('ADCMaxError');
      |       param.set('Enabled','off');
      |     end
      |   end
      | end
      mask DialogControl CompBut Prompt: Recalculate sample times
      mask DialogControl CompBut Tooltip: Simulink updates the sample times of all blocks when the simulation is run. This button will update the sample times now.
      mask DialogControl CompBut Callback:
      | btn=questdlg('This will apply all changes in all open dialog boxes and update the schematic. Do you want to proceed?','Apply all changes','Continue','Cancel','Continue');
      | if strcmp(btn,'Continue')
      |   dlgs=DAStudio.ToolRoot.getOpenDialogs;
      |   for i=1:length(dlgs)
      |     dlgs(i).apply;
      |   end
      |   try
      |     SampleTime_1=str2double(get_param(gcb,'SampleTime_1'));
      |     ts=Simulink.Block.getSampleTimes(gcb);
      |     ts=ts(1).Value(1);
      |     if (SampleTime_1 ~= ts)
      |       SampleTime_1=ts;
      |       set_param(gcb,'SampleTime_1',num2str(ts));
      |       autoCalcEn=get_param(gcb,'autoCalcEn');
      |       if strcmp(autoCalcEn,'on')
      |         SampleTime=Simulink.data.evalinGlobal(bdroot,get_param(gcb,'SampleTime'));
      |         p=Simulink.Mask.get(gcb);
      |         hintText=p.getDialogControl('timeHint');
      |         if SampleTime==-1
      |           SampleTime=SampleTime_1;
      |           hintText.Prompt='Caution: Implementation parameters depend on inherited sample time. Make sure that the sample time of the block''s inputs corresponds to the sampling period in the target application.';
      |         else
      |           hintText.Prompt='Caution: Implementation parameters depend on the sample time. Make sure that the simulation time step corresponds to the sampling period in the target application.';
      |         end
      |         fltADCMaxError_bkup=get_param(gcb,'fltADCMaxError');
      |         fltCC1sc_bkup=get_param(gcb,'fltCC1sc');
      |         fltCC2sc_bkup=get_param(gcb,'fltCC2sc');
      |         fltUpperLimit_bkup=get_param(gcb,'fltUpperLimit');
      |         fltLowerLimit_bkup=get_param(gcb,'fltLowerLimit');
      |         fltC1_bkup=get_param(gcb,'fltC1');
      |         if0=Simulink.data.evalinGlobal(bdroot,get_param(gcb,'if0'));
      |         iksi=Simulink.data.evalinGlobal(bdroot,get_param(gcb,'iksi'));
      |         ADCMaxError=Simulink.data.evalinGlobal(bdroot,get_param(gcb,'ADCMaxError'));
      |         if (if0<=0)
      |           warning('Natural frequency f0 must be positive.');
      |         end
      |         if (iksi<=0)
      |           warning('Feedback loop attenuation must be positive.');
      |         end
      |         if (iksi>1)
      |           warning('Feedback loop attenuation must not exceed 1.');
      |         end
      |         if (ADCMaxError<=0)
      |           warning('fltADCMaxError must be positive.');
      |         end
      |         fltADCMaxError=ADCMaxError;
      |         pgain=12.56637061435917*iksi*if0;
      |         igain=39.47841760435743*if0*if0;
      |         cc1=pgain+igain*SampleTime*0.5;
      |         cc2=-pgain+igain*SampleTime*0.5;
      |         fltCC1sc=cc1;
      |         fltCC2sc=cc2;
      |         fltLowerLimit=-1000000.0;
      |         fltUpperLimit=1000000.0;
      |         fltC1=SampleTime*0.5;
      |         if isnan(fltADCMaxError)
      |           if ~strcmp(fltADCMaxError_bkup,'0')
      |             set_param(gcb,'fltADCMaxError','0');
      |           end
      |         else
      |           tmps=num2str(fltADCMaxError);
      |           if ~strcmp(fltADCMaxError_bkup,tmps)
      |             set_param(gcb,'fltADCMaxError',tmps);
      |           end
      |         end
      |         if isnan(fltCC1sc)
      |           if ~strcmp(fltCC1sc_bkup,'0')
      |             set_param(gcb,'fltCC1sc','0');
      |           end
      |         else
      |           tmps=num2str(fltCC1sc);
      |           if ~strcmp(fltCC1sc_bkup,tmps)
      |             set_param(gcb,'fltCC1sc',tmps);
      |           end
      |         end
      |         if isnan(fltCC2sc)
      |           if ~strcmp(fltCC2sc_bkup,'0')
      |             set_param(gcb,'fltCC2sc','0');
      |           end
      |         else
      |           tmps=num2str(fltCC2sc);
      |           if ~strcmp(fltCC2sc_bkup,tmps)
      |             set_param(gcb,'fltCC2sc',tmps);
      |           end
      |         end
      |         if isnan(fltUpperLimit)
      |           if ~strcmp(fltUpperLimit_bkup,'0')
      |             set_param(gcb,'fltUpperLimit','0');
      |           end
      |         else
      |           tmps=num2str(fltUpperLimit);
      |           if ~strcmp(fltUpperLimit_bkup,tmps)
      |             set_param(gcb,'fltUpperLimit',tmps);
      |           end
      |         end
      |         if isnan(fltLowerLimit)
      |           if ~strcmp(fltLowerLimit_bkup,'0')
      |             set_param(gcb,'fltLowerLimit','0');
      |           end
      |         else
      |           tmps=num2str(fltLowerLimit);
      |           if ~strcmp(fltLowerLimit_bkup,tmps)
      |             set_param(gcb,'fltLowerLimit',tmps);
      |           end
      |         end
      |         if isnan(fltC1)
      |           if ~strcmp(fltC1_bkup,'0')
      |             set_param(gcb,'fltC1','0');
      |           end
      |         else
      |           tmps=num2str(fltC1);
      |           if ~strcmp(fltC1_bkup,tmps)
      |             set_param(gcb,'fltC1',tmps);
      |           end
      |         end
      |       end
      |     end
      |   catch
      |    warning(['Sample time cannot be calculated for the block ' gcb])
      |   end
      | end
      mask DialogControl timeHint Prompt: Note: Implementation parameters cannot be calculated yet because the block's inherited sample time is unknown. Simulink will update the sample time when you run the simulation.
      mask Display:
      | color('black');
      | pos = get_param(gcb, 'Position');
      | width = pos(3) - pos(1);
      | height = pos(4) - pos(2);
      | tX=width/2;
      | tY=height - 8;
      | color('black');
      | text(tX,tY, 'AMCLIB_Windmilling_FLT', 'horizontalAlignment', 'center');
      | if showStates == 2
      |   color('red');
      |   text(tX,tY - 20, ['debugging mode' char(13) char(10) '(limited performance)'], 'horizontalAlignment', 'center');
      | end
